simulink model "PD_digital_saturacao"  (R2019b)
settings: Solver=VariableStepAuto  StartTime=0.0  StopTime=7  RelTol=1e-3
settings Model: Creator=fernandopassold  LastModifiedBy=fernandopassold
settings DataIOCC: ReturnWorkspaceOutputs=off
settings DebuggingCC: ArithmeticOperatorsInVariantConditions=warning
settings SFSimCC: SimUseLocalCustomCode=off  CustomCodeUndefinedFunction=UseInterfaceOnly
settings RTWCC: RTWUseLocalCustomCode=off

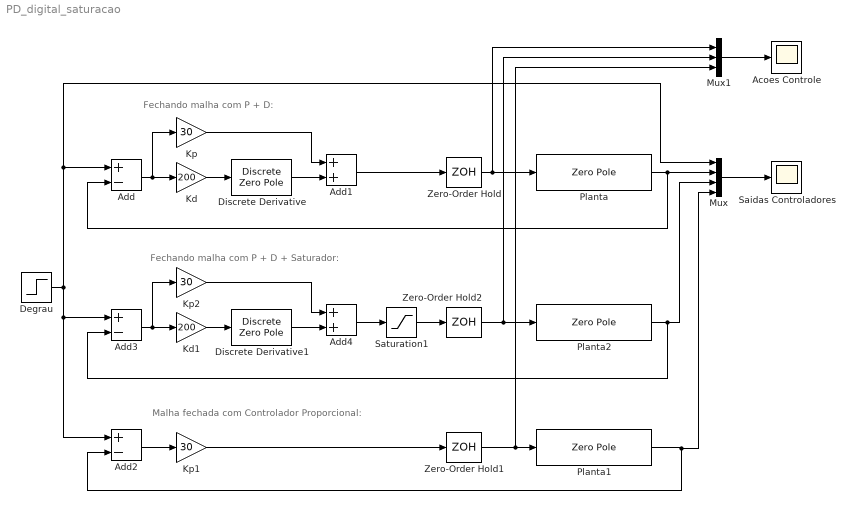
== system PD_digital_saturacao ==
  note: Fechando malha com P + D:
  note: Malha fechada com Controlador Proporcional:
  note: Fechando malha com P + D + Saturador:
  Acoes Controle : Scope
  Add : Sum  Inputs=+-
  Add1 : Sum
  Add2 : Sum  Inputs=+-
  Add3 : Sum  Inputs=+-
  Add4 : Sum
  Degrau : Step  SampleTime=0
  Discrete Derivative : DiscreteZeroPole  Poles=[0]  Gain=1  SampleTime=0.1
  Discrete Derivative1 : DiscreteZeroPole  Poles=[0]  Gain=1  SampleTime=0.1
  Kd : Gain  Gain=200
  Kd1 : Gain  Gain=200
  Kp : Gain  Gain=30
  Kp1 : Gain  Gain=30
  Kp2 : Gain  Gain=30
  Mux : Mux
  Mux1 : Mux  Inputs=3
  Planta : ZeroPole  Zeros=[ ]  Poles=[-1 -2 -10]
  Planta1 : ZeroPole  Zeros=[ ]  Poles=[-1 -2 -10]
  Planta2 : ZeroPole  Zeros=[ ]  Poles=[-1 -2 -10]
  Saidas Controladores : Scope
  Saturation1 : Saturate  UpperLimit=100  LowerLimit=0
  Zero-Order Hold : ZeroOrderHold  SampleTime=0.1
  Zero-Order Hold1 : ZeroOrderHold  SampleTime=0.1
  Zero-Order Hold2 : ZeroOrderHold  SampleTime=0.1
  wires:
  Planta/1 -> Add/2, Mux/2
  Zero-Order Hold/1 -> Mux1/1, Planta/1
  Add/1 -> Kd/1, Kp/1
  Discrete Derivative/1 -> Add1/2
  Kp/1 -> Add1/1
  Zero-Order Hold1/1 -> Mux1/3, Planta1/1
  Add2/1 -> Kp1/1
  Degrau/1 -> Add3/1, Add2/1, Mux/1, Add/1
  Kp1/1 -> Zero-Order Hold1/1
  Mux/1 -> Saidas Controladores/1
  Kd/1 -> Discrete Derivative/1
  Mux1/1 -> Acoes Controle/1
  Add1/1 -> Zero-Order Hold/1
  Kp2/1 -> Add4/1
  Kd1/1 -> Discrete Derivative1/1
  Add3/1 -> Kd1/1, Kp2/1
  Add4/1 -> Saturation1/1
  Saturation1/1 -> Zero-Order Hold2/1
  Planta2/1 -> Mux/3, Add3/2
  Discrete Derivative1/1 -> Add4/2
  Zero-Order Hold2/1 -> Mux1/2, Planta2/1
  Planta1/1 -> Mux/4, Add2/2
